simulink model "tests"  (R2021b)
settings: Solver=VariableStepAuto  StartTime=0.0  StopTime=1.99  MaxStep=1e-3  RelTol=1e-7
undefined symbols (not defined in the file): steel_roughness
settings Model: Creator=Ferran  LastModifiedBy=Ferran

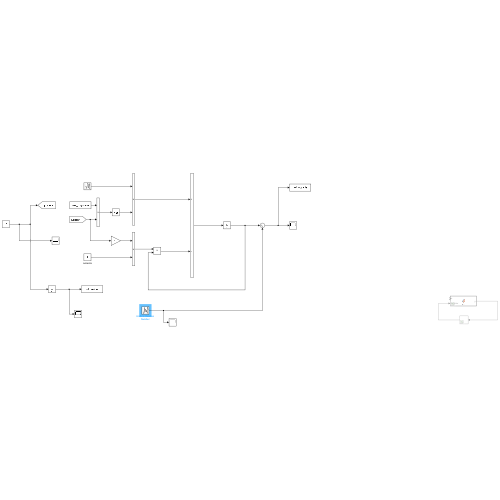
[thumbnail: Simulink's stored preview of the top-level diagram]
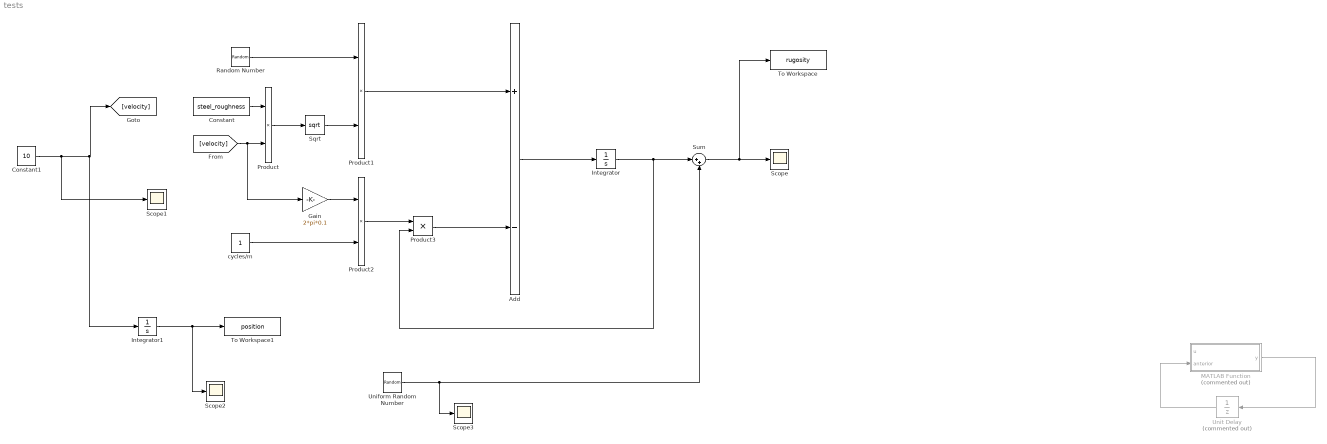
== system tests ==
  Add : Sum  Inputs=+-
  Constant : Constant  Value=steel_roughness
  Constant1 : Constant  Value=10
  Gain : Gain  Gain=2*pi*0.1
  Integrator : Integrator
  Integrator1 : Integrator
  MATLAB Function : MATLAB Function  Commented=on  TreatAsAtomicUnit=on
  Product{,1..3} (4 alike) : Product
  Random Number : RandomNumber  SampleTime=0.01
  Scope{,1..3} (4 alike) : Scope
  Sqrt : Sqrt  SaturateOnIntegerOverflow=on
  Sum : Sum  Inputs=|++
  To Workspace : ToWorkspace  VariableName=rugosity  SaveFormat=Timeseries  SampleTime=-1
  To Workspace1 : ToWorkspace  VariableName=position  SaveFormat=Timeseries  SampleTime=-1
  Uniform Random Number : UniformRandomNumber  Minimum=-2e-3  Maximum=2e-3  SampleTime=2/10
  Unit Delay : UnitDelay  Commented=on  SampleTime=-1  HasFrameUpgradeWarning=on
  cycles/m : Constant
  wires:
  Random Number/1 -> Product1/1
  Constant/1 -> Product/1
  [velocity] -> Gain/1, Product/2
  Product/1 -> Sqrt/1
  Sqrt/1 -> Product1/2
  Gain/1 -> Product2/1
  cycles/m/1 -> Product2/2
  Product1/1 -> Add/1
  Add/1 -> Integrator/1
  Integrator/1 -> Product3/2, Sum/1
  Product2/1 -> Product3/1
  Product3/1 -> Add/2
  Sum/1 -> To Workspace/1, Scope/1
  Constant1/1 -> Scope1/1, Integrator1/1, [velocity]
  Integrator1/1 -> Scope2/1, To Workspace1/1
  Unit Delay/1 -> MATLAB Function/2(anterior)
  MATLAB Function/1(y) -> Unit Delay/1
  Uniform Random Number/1 -> Scope3/1, Sum/2

== matlab function tests/MATLAB Function ==
  data: u input; y output; anterior input
function y = fcn(u, anterior)

r = -3 + 6*rand(1,1);

if u == 0
    y = 0;
elseif mod(u,2) == 0
    y = anterior + r;
else
    y = anterior;
end
